simulink model "buck_converter_open_loop_model"  (R2019a)
settings: Solver=VariableStepAuto  StartTime=0.0  StopTime=0.1  MaxStep=1e-5  RelTol=1e-5
values from neighbouring files (symbols this model uses):
  C = 68e-6    (= 6.8e-05)    [parameters_open_loop_with_various_load.m]
  Duty = (V/Vg)*(1+((RL+Rdson)/R))    (= 0.2650416)    [parameters_open_loop_with_various_load.m]
  L = 68e-6    (= 6.8e-05)    [parameters_open_loop_with_various_load.m]
  R = V/I    (= 0.36036036036)    [parameters_open_loop_with_various_load.m]
  Resr = 9e-3    (= 0.009)    [parameters_open_loop_with_various_load.m]
  RL = 30e-3    (= 0.03)    [parameters_open_loop_with_various_load.m]
  Vg = 5    [parameters_open_loop_with_various_load.m]
  Vm = 5    [parameters_open_loop_with_various_load.m]
libraries: powerlib x19, simulink x1
settings Model: Creator=Görkem  LastModifiedBy=Görkem

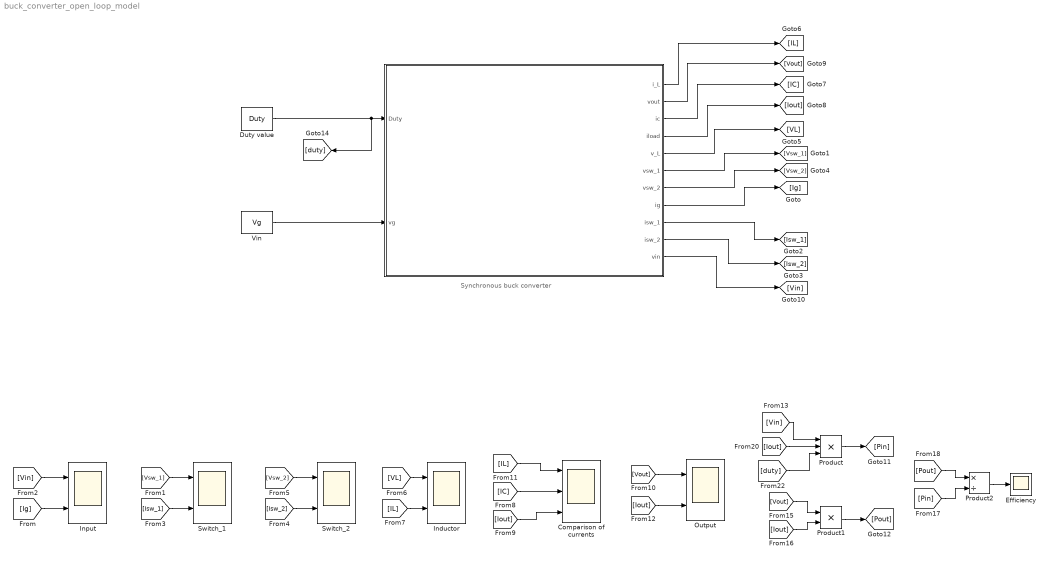
== system buck_converter_open_loop_model ==
  note: Synchronous buck converter
  "   " : Subsystem
  Comparison of currents : Scope  NumInputPorts=3
  Duty value : Constant  Value=Duty
  Efficiency : Scope
  Inductor : Scope  NumInputPorts=2
  Input : Scope  NumInputPorts=2
  "Output " : Scope  NumInputPorts=2
  Product : Product  Inputs=3
  Product1 : Product
  Product2 : Product  Inputs=*/
  Switch_1 : Scope  NumInputPorts=2
  Switch_2 : Scope  NumInputPorts=2
  Vin : Constant  Value=Vg
  wires:
  [Vsw_1] -> Switch_1/1
  [Isw_1] -> Switch_1/2
  [Vsw_2] -> Switch_2/1
  [Isw_2] -> Switch_2/2
  [VL] -> Inductor/1
  [IL] -> Inductor/2
  [IL] -> Comparison of currents/1
  [IC] -> Comparison of currents/2
  [Iout] -> Comparison of currents/3
  [Vout] -> "Output "/1
  [Iout] -> "Output "/2
  [Vin] -> Input/1
  [Ig] -> Input/2
  [Vin] -> Product/1
  [Iout] -> Product/2
  [Vout] -> Product1/1
  [Iout] -> Product1/2
  Product1/1 -> [Pout]
  Product/1 -> [Pin]
  [Pout] -> Product2/1
  [Pin] -> Product2/2
  Product2/1 -> Efficiency/1
  [duty] -> Product/3
  Duty value/1 -> [duty], "   "/1(Duty)
  "   "/4(iload) -> [Iout]
  "   "/3(ic) -> [IC]
  "   "/2(vout) -> [Vout]
  "   "/1(i_L) -> [IL]
  "   "/5(v_L) -> [VL]
  "   "/6(vsw_1) -> [Vsw_1]
  "   "/7(vsw_2) -> [Vsw_2]
  "   "/8(ig) -> [Ig]
  "   "/9(isw_1) -> [Isw_1]
  "   "/10(isw_2) -> [Isw_2]
  "   "/11(vin) -> [Vin]
  Vin/1 -> "   "/2(vg)

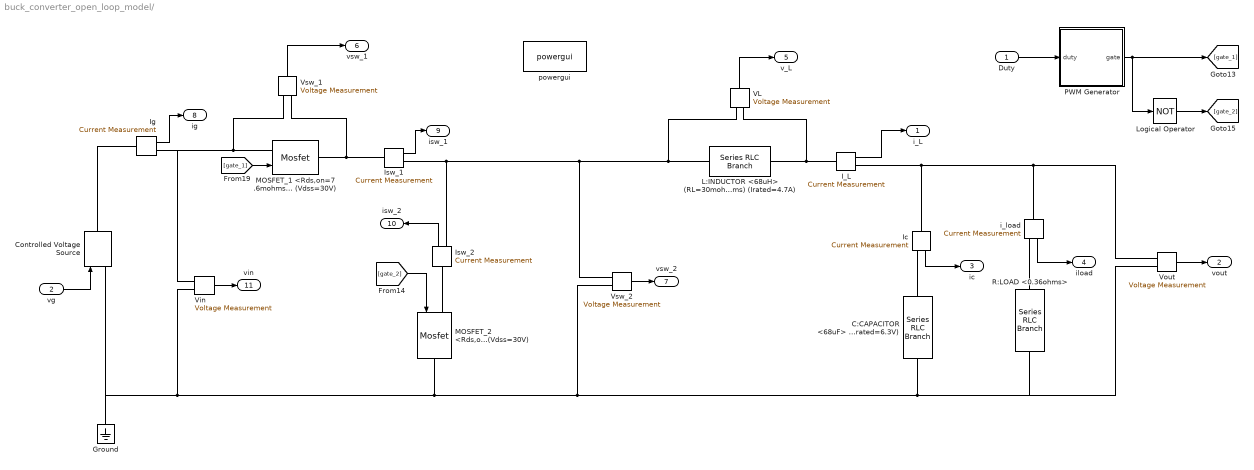
== system buck_converter_open_loop_model/    ==
  Duty : Inport
  vg : Inport  Port=2
  C:CAPACITOR <68uF> (Resr=9mohms) (Vrated=6.3V) : powerlib/Elements/Series RLC Branch  LConnTagsString=__new0  RConnTagsString=__new0  BranchType=RC  Resistance=Resr  Inductance=1e-3  SetiL0=off  InitialCurrent=0  Capacitance=C  Setx0=off  InitialVoltage=0  Measurements=None
      settings: SourceProductName=Simscape Electrical
  Controlled Voltage Source : powerlib/Electrical Sources/Controlled Voltage Source  Initialize=on  Source_Type=DC  Amplitude=0  Phase=0  Frequency=0  Measurements=None
      settings: SourceProductName=Simscape Electrical
  Ground : powerlib/Elements/Ground  LConnTagsString=a
      settings: SourceProductName=Simscape Electrical
  I_L : powerlib/Measurements/Current Measurement  PhasorSimulation=off  OutputType=Complex  PSBequivalent=0
      settings: SourceProductName=Simscape Electrical
  Ic : powerlib/Measurements/Current Measurement  PhasorSimulation=off  OutputType=Complex  PSBequivalent=0
      settings: SourceProductName=Simscape Electrical
  Ig : powerlib/Measurements/Current Measurement  PhasorSimulation=off  OutputType=Complex  PSBequivalent=0
      settings: SourceProductName=Simscape Electrical
  Isw_1 : powerlib/Measurements/Current Measurement  PhasorSimulation=off  OutputType=Complex  PSBequivalent=0
      settings: SourceProductName=Simscape Electrical
  Isw_2 : powerlib/Measurements/Current Measurement  PhasorSimulation=off  OutputType=Complex  PSBequivalent=0
      settings: SourceProductName=Simscape Electrical
  "L:INDUCTOR <68uH> (RL=30mohms) (Irated=4.7A) " : powerlib/Elements/Series RLC Branch  LConnTagsString=__new0  RConnTagsString=__new0  BranchType=RL  Resistance=RL  Inductance=L  SetiL0=off  InitialCurrent=0  Capacitance=1e-6  Setx0=off  InitialVoltage=0  Measurements=None
      settings: SourceProductName=Simscape Electrical
  Logical Operator : Logic  Operator=NOT  AllPortsSameDT=off  OutDataTypeStr=boolean
  MOSFET_1 <Rds,on=7.6mohms> (Ids=7A) (Vdss=30V) : powerlib/Power Electronics/Mosfet  Ron=Rdson  Lon=0  Rd=0  Vfd=Vf  IC=0  Rs=1e5  Cs=inf  Measurements=off
      settings: SourceProductName=Simscape Electrical
  MOSFET_2 <Rds,on=7.6mohms> (Ids=7A) (Vdss=30V) : powerlib/Power Electronics/Mosfet  Ron=Rdson  Lon=0  Rd=0  Vfd=Vf  IC=0  Rs=1e5  Cs=inf  Measurements=off
      settings: SourceProductName=Simscape Electrical
  PWM Generator : Subsystem
  "R:LOAD <0.36ohms> " : powerlib/Elements/Series RLC Branch  LConnTagsString=__new0  RConnTagsString=__new0  BranchType=R  Resistance=R  Inductance=1e-3  SetiL0=off  InitialCurrent=0  Capacitance=47e-6  Setx0=off  InitialVoltage=0  Measurements=None
      settings: SourceProductName=Simscape Electrical
  VL : powerlib/Measurements/Voltage Measurement  PhasorSimulation=off  OutputType=Complex  PSBequivalent=0
      settings: SourceProductName=Simscape Electrical
  Vin : powerlib/Measurements/Voltage Measurement  PhasorSimulation=off  OutputType=Complex  PSBequivalent=0
      settings: SourceProductName=Simscape Electrical
  Vout : powerlib/Measurements/Voltage Measurement  PhasorSimulation=off  OutputType=Complex  PSBequivalent=0
      settings: SourceProductName=Simscape Electrical
  Vsw_1 : powerlib/Measurements/Voltage Measurement  PhasorSimulation=off  OutputType=Complex  PSBequivalent=0
      settings: SourceProductName=Simscape Electrical
  Vsw_2 : powerlib/Measurements/Voltage Measurement  PhasorSimulation=off  OutputType=Complex  PSBequivalent=0
      settings: SourceProductName=Simscape Electrical
  i_load : powerlib/Measurements/Current Measurement  PhasorSimulation=off  OutputType=Complex  PSBequivalent=0
      settings: SourceProductName=Simscape Electrical
  powergui : powerlib/powergui  Priority=1  SimulationMode=Continuous  SampleTime=50e-6  frequency=60  Iterations=50  frequencyindice=0  Pbase=100e6  ErrMax=1e-4  UnitsV=kV  UnitsW=MW  buscounter=0  FunctionMessages=off  echomessages=off  EnableUseOfTLC=off  CurrentSourceSwitches=off  DisableSnubberDevices=off  DisableRonSwitches=off  DisableVfSwitches=off  DisplayEquations=off  AutomaticDiscreteSolvers=off  SolverType=Tustin/Backward Euler (TBE)  Interpol=off  ExternalGateDelay=off  methode=off  Ts=100  x0status=blocks  SPID=on  SwTol=0  HookPort=off  NonlinearTolerance=0  nMaxIteration=15  ContinueOnMaxIteration=off  RestoreLinks=warning  ResistiveCurrentMeasurement=off  Frange=[0:2:500]  Ylog=off  Xlog=on  ShowGrid=off  save=off  variable=ZData  structure=0  ZoomFFT=off  StartTime=0.0  cycles=1  DisplayStyle=1  fundamental=60  FreqAxis=off  MaxFrequency=1000  frequencyindicesteady=1  RmsSteady=1  display=off
      settings: SourceProductName=Simscape Electrical
  i_L : Outport
  vout : Outport  Port=2
  ic : Outport  Port=3
  iload : Outport  Port=4
  v_L : Outport  Port=5
  vsw_1 : Outport  Port=6
  vsw_2 : Outport  Port=7
  ig : Outport  Port=8
  isw_1 : Outport  Port=9
  isw_2 : Outport  Port=10
  vin : Outport  Port=11
  wires:
  Logical Operator/1 -> [gate_2]
  Duty/1 -> PWM Generator/1(duty)
  [gate_2] -> MOSFET_2 <Rds,on=7.6mohms> (Ids=7A) (Vdss=30V)/1
  i_load/1 -> iload/1
  Vout/1 -> vout/1
  I_L/1 -> i_L/1
  Ic/1 -> ic/1
  Vsw_2/1 -> vsw_2/1
  [gate_1] -> MOSFET_1 <Rds,on=7.6mohms> (Ids=7A) (Vdss=30V)/1
  PWM Generator/1(gate) -> Logical Operator/1, [gate_1]
  Ig/1 -> ig/1
  Isw_1/1 -> isw_1/1
  VL/1 -> v_L/1
  Isw_2/1 -> isw_2/1
  Vin/1 -> vin/1
  Vsw_1/1 -> vsw_1/1
  vg/1 -> Controlled Voltage Source/1
  connections:
  MOSFET_1 <Rds,on=7.6mohms> (Ids=7A) (Vdss=30V)/LConn1 -- Vin/LConn1 -- Ig/RConn1 -- Vsw_1/LConn1
  Controlled Voltage Source/LConn1 -- Ground/LConn1 -- Vin/LConn2 -- Vsw_2/LConn2 -- Vout/LConn2 -- "R:LOAD <0.36ohms> "/RConn1 -- C:CAPACITOR <68uF> (Resr=9mohms) (Vrated=6.3V)/RConn1 -- MOSFET_2 <Rds,on=7.6mohms> (Ids=7A) (Vdss=30V)/RConn1
  Isw_1/RConn1 -- Isw_2/RConn1 -- Vsw_2/LConn1 -- "L:INDUCTOR <68uH> (RL=30mohms) (Irated=4.7A) "/LConn1 -- VL/LConn1
  I_L/RConn1 -- i_load/LConn1 -- Vout/LConn1 -- Ic/LConn1
  Controlled Voltage Source/RConn1 -- Ig/LConn1
  I_L/LConn1 -- VL/LConn2 -- "L:INDUCTOR <68uH> (RL=30mohms) (Irated=4.7A) "/RConn1
  Vsw_1/LConn2 -- Isw_1/LConn1 -- MOSFET_1 <Rds,on=7.6mohms> (Ids=7A) (Vdss=30V)/RConn1
  MOSFET_2 <Rds,on=7.6mohms> (Ids=7A) (Vdss=30V)/LConn1 -- Isw_2/LConn1
  Ic/RConn1 -- C:CAPACITOR <68uF> (Resr=9mohms) (Vrated=6.3V)/LConn1
  i_load/RConn1 -- "R:LOAD <0.36ohms> "/LConn1

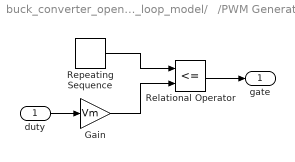
== system buck_converter_open_loop_model/   /PWM Generator ==
  duty : Inport
  Gain : Gain  Gain=Vm
  Relational Operator : RelationalOperator  Operator=<=  OutDataTypeStr=boolean  RndMeth=Simplest
  Repeating Sequence : simulink/Sources/Repeating Sequence  rep_seq_t=[0 0.5/50000 1/50000]  rep_seq_y=[0 Vm 0]
  gate : Outport
  wires:
  Repeating Sequence/1 -> Relational Operator/1
  Relational Operator/1 -> gate/1
  duty/1 -> Gain/1
  Gain/1 -> Relational Operator/2
